simulink model "Modelo_3_masas"  (R2020b)
settings: Solver=VariableStepAuto  StartTime=0.0  StopTime=20  RelTol=1e-3
undefined symbols (not defined in the file): sigbuilder_block
settings Model: Creator=Marce  LastModifiedBy=Marce

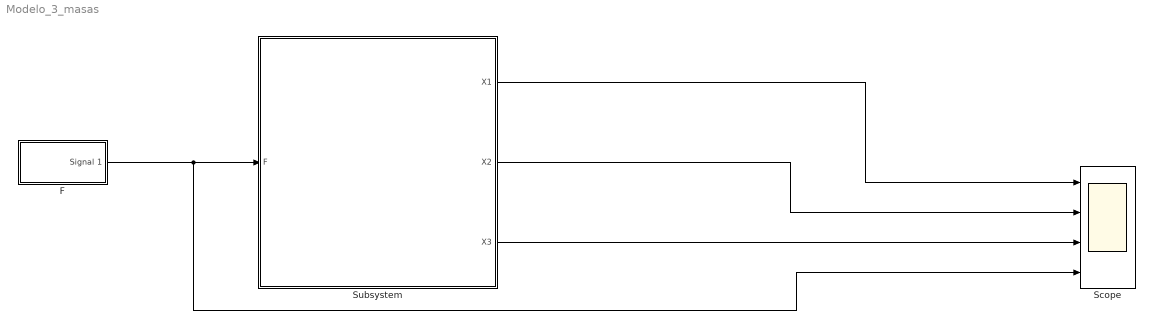
== system Modelo_3_masas ==
  F : Subsystem  Tag=STV Subsys  LoadFcn=sigbuilder_block('load');  StartFcn=sigbuilder_block('start');  StopFcn=sigbuilder_block('stop');  ClipboardFcn=sigbuilder_block('clipboard');  mask(Sigbuilder block){tuvar=[0:10]}
      mask help: Simulink:masks:SigbuilderBlock_MD
      mask init:
      | if ~strcmp(get_param(bdroot(gcbh),'SimulationStatus'),'stopped') tuvar = sigbuilder_block('maskInit'); end
      settings: CopyFcn=sigbuilder_block('copy');  DeleteFcn=sigbuilder_block('delete');  ModelCloseFcn=sigbuilder_block('modelClose');  PreSaveFcn=sigbuilder_block('preSave');  PauseFcn=sigbuilder_block('pause');  ContinueFcn=sigbuilder_block('continue');  NameChangeFcn=sigbuilder_block('namechange');  OpenFcn=sigbuilder_block('open',[403.5 153 550.5 359.25 ]);  CloseFcn=sigbuilder_block('close');
      mask Display: plot(0, 0, 100, 100,[2, 2, 32, 32, 2], [68, 8, 8, 68, 68],[32, 2], [38, 38], [32, 19, 2],[53, 60, 44], [32, 17, 17, 2],[16, 16, 31, 31]);txt = getActiveGroup(gcbh);text(2, 100, txt,'verticalAlignment', 'top');
  Scope : Scope  NumInputPorts=4
  Subsystem : Subsystem
  wires:
  F/1(Signal 1) -> Subsystem/1(F), Scope/4
  Subsystem/1(X1) -> Scope/1
  Subsystem/2(X2) -> Scope/2
  Subsystem/3(X3) -> Scope/3

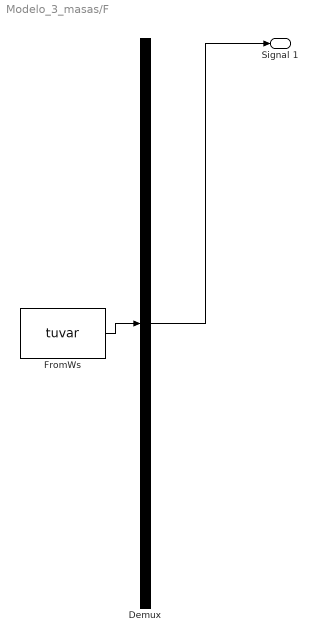
== system Modelo_3_masas/F ==
  Demux : Demux  Tag=STV Demux  Outputs=1
      settings: DisplayOption=none
  FromWs : FromWorkspace  Tag=STV FromWs  VariableName=tuvar
      SigBuilderData=|
      | common.afterFinalStr = 'Extrapolate'
      | common.sampleTime = 0
      | dataSet.timeRange = [0 10]
      | dataSet.name = 'Group 1'
      | sbobj.Groups.Name = 'Group 1'
      | sbobj.Groups.Signals.Name = 'Signal 1'
      | sbobj.Groups.Signals.XData = [0 4 4 6 6 10]
      | sbobj.Groups.Signals.YData = [0 0 1 1 0 0]
  Signal 1 : Outport  Tag=STV Outport
  wires:
  Demux/1 -> Signal 1/1
  FromWs/1 -> Demux/1

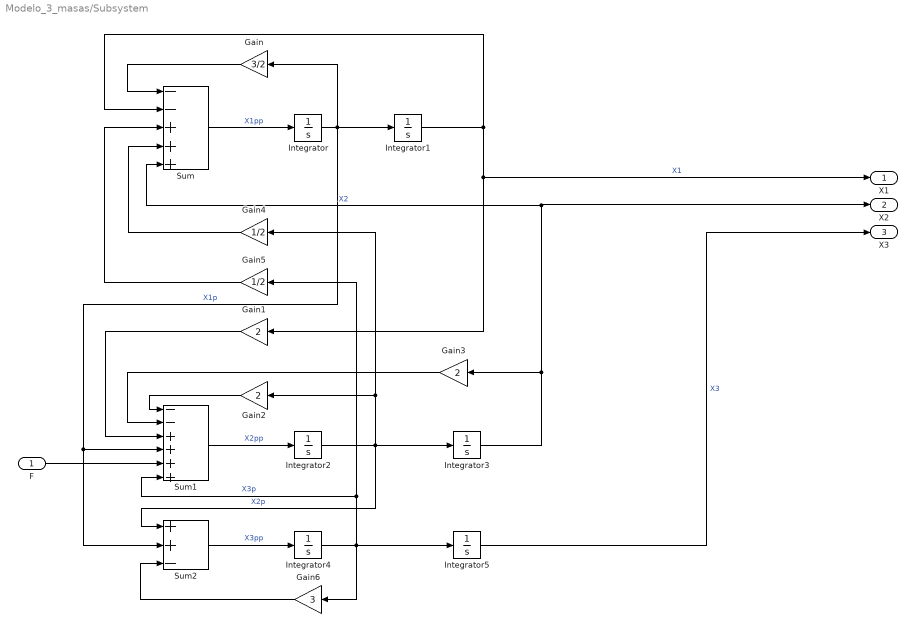
== system Modelo_3_masas/Subsystem ==
  F : Inport
  Gain : Gain  Gain=3/2
  Gain1 : Gain  Gain=2
  Gain2 : Gain  Gain=2
  Gain3 : Gain  Gain=2
  Gain4 : Gain  Gain=1/2
  Gain5 : Gain  Gain=1/2
  Gain6 : Gain  Gain=3
  Integrator{,1..5} (6 alike) : Integrator
  Sum : Sum  Inputs=--+++
  Sum1 : Sum  Inputs=--++++
  Sum2 : Sum  Inputs=++-
  X1 : Outport
  X2 : Outport  Port=2
  X3 : Outport  Port=3
  wires:
  Integrator2/1 -> Sum2/1, Gain2/1, Gain4/1, Integrator3/1  "X2p"
  Integrator1/1 -> X1/1, Gain1/1, Sum/2  "X1"
  Gain5/1 -> Sum/3
  Gain3/1 -> Sum1/2
  Integrator/1 -> Sum2/2, Sum1/4, Gain/1, Integrator1/1  "X1p"
  Gain2/1 -> Sum1/1
  Gain1/1 -> Sum1/3
  Integrator3/1 -> X2/1, Sum/5, Gain3/1  "X2"
  Sum/1 -> Integrator/1  "X1pp"
  Integrator4/1 -> Gain6/1, Sum1/6, Gain5/1, Integrator5/1  "X3p"
  Sum1/1 -> Integrator2/1  "X2pp"
  Sum2/1 -> Integrator4/1  "X3pp"
  Gain/1 -> Sum/1
  Gain6/1 -> Sum2/3
  Gain4/1 -> Sum/4
  Integrator5/1 -> X3/1  "X3"
  F/1 -> Sum1/5
